simulink model "REL"  (R2022a)
settings: Solver=FixedStepDiscrete  StartTime=0.0  StopTime=10.0  FixedStep=0.01  RelTol=1e-3
libraries: simulink x4, DoorRatSts x4, DoorRlsDriver x2, DoorRlsReq x2
settings Model: Creator=DELL  LastModifiedBy=DELL
settings DataIOCC: SaveFormat=StructureWithTime
settings OptimizationCC: DefaultParameterBehavior=Inlined  EnhancedBackFolding=on  PassReuseOutputArgsAs=Individual arguments  ZeroExternalMemoryAtStartup=off  ZeroInternalMemoryAtStartup=off  OptimizeBlockOrder=speed  DifferentSizesBufferReuse=on  OptimizationCustomize=off  EfficientTunableParamExpr=on
settings DebuggingCC: ParameterTunabilityLossMsg=error
settings ModelReferenceCC: ModelReferenceNumInstancesAllowed=Single
settings SFSimCC: MATLABDynamicMemAlloc=off
settings RTWCC: Description=AUTOSAR  SystemTargetFile=autosar.tlc  GenCodeOnly=on  TemplateMakefile=ert_default_tmf
settings CodeAppCC: ForceParamTrailComments=on  IgnoreCustomStorageClasses=off  OperatorAnnotations=on  SimulinkDataObjDesc=on  SFDataObjDesc=on  InsertBlockDesc=on
settings STFCustomTargetCC: TargetLangStandard=C99 (ISO)  MultiwordLength=256  ParMdlRefBuildCompliant=on  CompOptLevelCompliant=on  IncludeMdlTerminateFcn=off  CombineOutputUpdateFcns=on  SuppressErrorStatus=on  ERTCustomFileBanners=on  SupportNonFinite=off  SupportComplex=off  SupportContinuousTime=off  SupportNonInlinedSFcns=off  RemoveResetFunc=on  MATLABClassNameForMDSCustomization=Simulink.SoftwareTarget.ERTCustomization  AutosarCompliant=on  GRTInterface=off  UseToolchainInfoCompliant=on  LookupTableObjectStructAxisOrder=2,1,3,4,...  LUTObjectStructOrderEvenSpacing=Size,Table,Breakpoints  SystemTargetFile=autosar.tlc
settings ERTTargetCC: TargetLangStandard=C99 (ISO)  ConcurrentExecutionCompliant=off  IncludeMdlTerminateFcn=off  SuppressErrorStatus=on  SupportNonFinite=off  SupportComplex=off  ModelStepFunctionPrototypeControlCompliant=off  CPPClassGenCompliant=off  AutosarCompliant=on  LookupTableObjectStructAxisOrder=2,1,3,4,...  LUTObjectStructOrderEvenSpacing=Size,Table,Breakpoints  InlinedParameterPlacement=NonHierarchical  ERTCustomFileTemplate=example_file_process.tlc

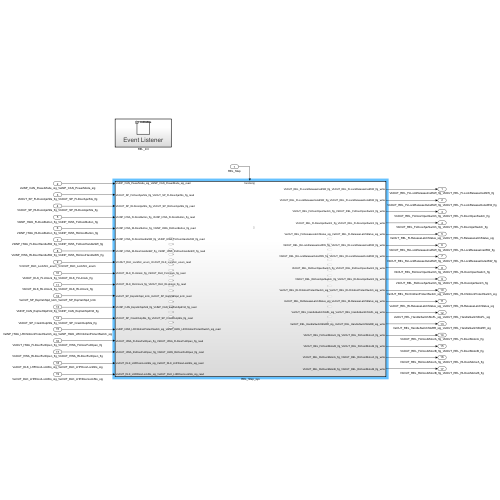
[thumbnail: Simulink's stored preview of the top-level diagram]
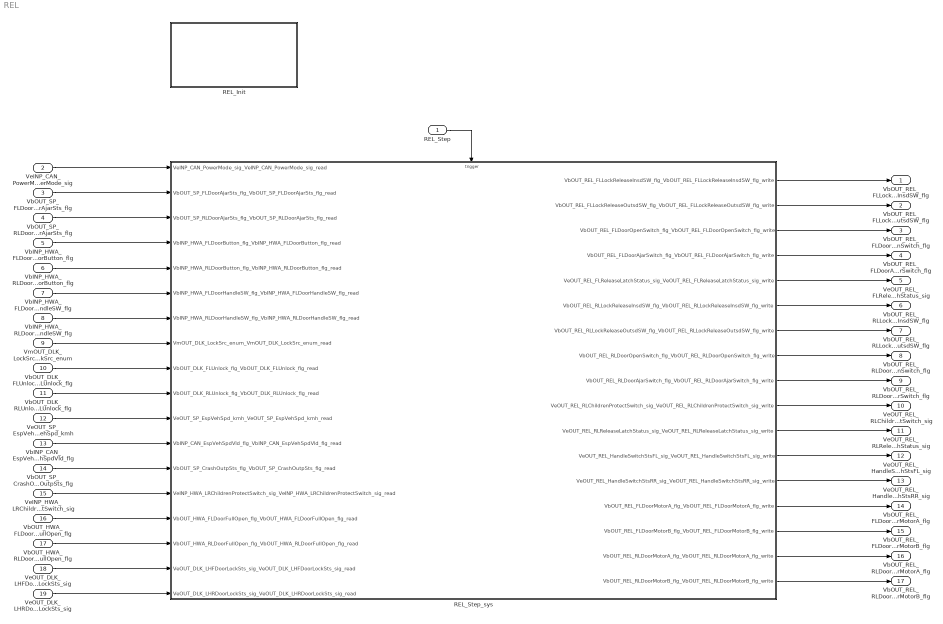
== system REL ==
  REL_Step : Inport  SampleTime=0.01  OutputFunctionCall=on
  VeINP_CAN_PowerMode_sig_VeINP_CAN_PowerMode_sig : Inport  Port=2  OutDataTypeStr=UInt8  PortDimensions=1
  VbOUT_SP_FLDoorAjarSts_flg_VbOUT_SP_FLDoorAjarSts_flg : Inport  Port=3  OutDataTypeStr=Boolean  PortDimensions=1
  VbOUT_SP_RLDoorAjarSts_flg_VbOUT_SP_RLDoorAjarSts_flg : Inport  Port=4  OutDataTypeStr=Boolean  PortDimensions=1
  VbINP_HWA_FLDoorButton_flg_VbINP_HWA_FLDoorButton_flg : Inport  Port=5  OutDataTypeStr=Boolean  PortDimensions=1
  VbINP_HWA_RLDoorButton_flg_VbINP_HWA_RLDoorButton_flg : Inport  Port=6  OutDataTypeStr=Boolean  PortDimensions=1
  VbINP_HWA_FLDoorHandleSW_flg_VbINP_HWA_FLDoorHandleSW_flg : Inport  Port=7  OutDataTypeStr=Boolean  PortDimensions=1
  VbINP_HWA_RLDoorHandleSW_flg_VbINP_HWA_RLDoorHandleSW_flg : Inport  Port=8  OutDataTypeStr=Boolean  PortDimensions=1
  VmOUT_DLK_LockSrc_enum_VmOUT_DLK_LockSrc_enum : Inport  Port=9  OutDataTypeStr=UInt8  PortDimensions=1
  VbOUT_DLK_FLUnlock_flg_VbOUT_DLK_FLUnlock_flg : Inport  Port=10  OutDataTypeStr=Boolean  PortDimensions=1
  VbOUT_DLK_RLUnlock_flg_VbOUT_DLK_RLUnlock_flg : Inport  Port=11  OutDataTypeStr=Boolean  PortDimensions=1
  VeOUT_SP_EspVehSpd_kmh_VeOUT_SP_EspVehSpd_kmh : Inport  Port=12  OutDataTypeStr=UInt8  PortDimensions=1
  VbINP_CAN_EspVehSpdVld_flg_VbINP_CAN_EspVehSpdVld_flg : Inport  Port=13  OutDataTypeStr=Boolean  PortDimensions=1
  VbOUT_SP_CrashOutpSts_flg_VbOUT_SP_CrashOutpSts_flg : Inport  Port=14  OutDataTypeStr=Boolean  PortDimensions=1
  VeINP_HWA_LRChildrenProtectSwitch_sig_VeINP_HWA_LRChildrenProtectSwitch_sig : Inport  Port=15  OutDataTypeStr=UInt8  PortDimensions=1
  VbOUT_HWA_FLDoorFullOpen_flg_VbOUT_HWA_FLDoorFullOpen_flg : Inport  Port=16  OutDataTypeStr=Boolean  PortDimensions=1
  VbOUT_HWA_RLDoorFullOpen_flg_VbOUT_HWA_RLDoorFullOpen_flg : Inport  Port=17  OutDataTypeStr=Boolean  PortDimensions=1
  VeOUT_DLK_LHFDoorLockSts_sig_VeOUT_DLK_LHFDoorLockSts_sig : Inport  Port=18  OutDataTypeStr=UInt8  PortDimensions=1
  VeOUT_DLK_LHRDoorLockSts_sig_VeOUT_DLK_LHRDoorLockSts_sig : Inport  Port=19  OutDataTypeStr=UInt8  PortDimensions=1
  REL_Init : Subsystem
  REL_Step_sys : Subsystem
  VbOUT_REL_FLLockReleaseInsdSW_flg_VbOUT_REL_FLLockReleaseInsdSW_flg : Outport  OutDataTypeStr=Boolean  PortDimensions=1
  VbOUT_REL_FLLockReleaseOutsdSW_flg_VbOUT_REL_FLLockReleaseOutsdSW_flg : Outport  Port=2  OutDataTypeStr=Boolean  PortDimensions=1
  VbOUT_REL_FLDoorOpenSwitch_flg_VbOUT_REL_FLDoorOpenSwitch_flg : Outport  Port=3  OutDataTypeStr=Boolean  PortDimensions=1
  VbOUT_REL_FLDoorAjarSwitch_flg_VbOUT_REL_FLDoorAjarSwitch_flg : Outport  Port=4  OutDataTypeStr=Boolean  PortDimensions=1
  VeOUT_REL_FLReleaseLatchStatus_sig_VeOUT_REL_FLReleaseLatchStatus_sig : Outport  Port=5  OutDataTypeStr=UInt8  PortDimensions=1
  VbOUT_REL_RLLockReleaseInsdSW_flg_VbOUT_REL_RLLockReleaseInsdSW_flg : Outport  Port=6  OutDataTypeStr=Boolean  PortDimensions=1
  VbOUT_REL_RLLockReleaseOutsdSW_flg_VbOUT_REL_RLLockReleaseOutsdSW_flg : Outport  Port=7  OutDataTypeStr=Boolean  PortDimensions=1
  VbOUT_REL_RLDoorOpenSwitch_flg_VbOUT_REL_RLDoorOpenSwitch_flg : Outport  Port=8  OutDataTypeStr=Boolean  PortDimensions=1
  VbOUT_REL_RLDoorAjarSwitch_flg_VbOUT_REL_RLDoorAjarSwitch_flg : Outport  Port=9  OutDataTypeStr=Boolean  PortDimensions=1
  VeOUT_REL_RLChildrenProtectSwitch_sig_VeOUT_REL_RLChildrenProtectSwitch_sig : Outport  Port=10  OutDataTypeStr=UInt8  PortDimensions=1
  VeOUT_REL_RLReleaseLatchStatus_sig_VeOUT_REL_RLReleaseLatchStatus_sig : Outport  Port=11  OutDataTypeStr=UInt8  PortDimensions=1
  VeOUT_REL_HandleSwitchStsFL_sig_VeOUT_REL_HandleSwitchStsFL_sig : Outport  Port=12  OutDataTypeStr=UInt8  PortDimensions=1
  VeOUT_REL_HandleSwitchStsRR_sig_VeOUT_REL_HandleSwitchStsRR_sig : Outport  Port=13  OutDataTypeStr=UInt8  PortDimensions=1
  VbOUT_REL_FLDoorMotorA_flg_VbOUT_REL_FLDoorMotorA_flg : Outport  Port=14  OutDataTypeStr=Boolean  PortDimensions=1
  VbOUT_REL_FLDoorMotorB_flg_VbOUT_REL_FLDoorMotorB_flg : Outport  Port=15  OutDataTypeStr=Boolean  PortDimensions=1
  VbOUT_REL_RLDoorMotorA_flg_VbOUT_REL_RLDoorMotorA_flg : Outport  Port=16  OutDataTypeStr=Boolean  PortDimensions=1
  VbOUT_REL_RLDoorMotorB_flg_VbOUT_REL_RLDoorMotorB_flg : Outport  Port=17  OutDataTypeStr=Boolean  PortDimensions=1
  wires:
  VeINP_CAN_PowerMode_sig_VeINP_CAN_PowerMode_sig/1 -> REL_Step_sys/1(VeINP_CAN_PowerMode_sig_VeINP_CAN_PowerMode_sig_read)
  VbOUT_SP_FLDoorAjarSts_flg_VbOUT_SP_FLDoorAjarSts_flg/1 -> REL_Step_sys/2(VbOUT_SP_FLDoorAjarSts_flg_VbOUT_SP_FLDoorAjarSts_flg_read)
  VbOUT_SP_RLDoorAjarSts_flg_VbOUT_SP_RLDoorAjarSts_flg/1 -> REL_Step_sys/3(VbOUT_SP_RLDoorAjarSts_flg_VbOUT_SP_RLDoorAjarSts_flg_read)
  VbINP_HWA_FLDoorButton_flg_VbINP_HWA_FLDoorButton_flg/1 -> REL_Step_sys/4(VbINP_HWA_FLDoorButton_flg_VbINP_HWA_FLDoorButton_flg_read)
  VbINP_HWA_RLDoorButton_flg_VbINP_HWA_RLDoorButton_flg/1 -> REL_Step_sys/5(VbINP_HWA_RLDoorButton_flg_VbINP_HWA_RLDoorButton_flg_read)
  VbINP_HWA_FLDoorHandleSW_flg_VbINP_HWA_FLDoorHandleSW_flg/1 -> REL_Step_sys/6(VbINP_HWA_FLDoorHandleSW_flg_VbINP_HWA_FLDoorHandleSW_flg_read)
  VbINP_HWA_RLDoorHandleSW_flg_VbINP_HWA_RLDoorHandleSW_flg/1 -> REL_Step_sys/7(VbINP_HWA_RLDoorHandleSW_flg_VbINP_HWA_RLDoorHandleSW_flg_read)
  VmOUT_DLK_LockSrc_enum_VmOUT_DLK_LockSrc_enum/1 -> REL_Step_sys/8(VmOUT_DLK_LockSrc_enum_VmOUT_DLK_LockSrc_enum_read)
  VbOUT_DLK_FLUnlock_flg_VbOUT_DLK_FLUnlock_flg/1 -> REL_Step_sys/9(VbOUT_DLK_FLUnlock_flg_VbOUT_DLK_FLUnlock_flg_read)
  VbOUT_DLK_RLUnlock_flg_VbOUT_DLK_RLUnlock_flg/1 -> REL_Step_sys/10(VbOUT_DLK_RLUnlock_flg_VbOUT_DLK_RLUnlock_flg_read)
  VeOUT_SP_EspVehSpd_kmh_VeOUT_SP_EspVehSpd_kmh/1 -> REL_Step_sys/11(VeOUT_SP_EspVehSpd_kmh_VeOUT_SP_EspVehSpd_kmh_read)
  VbINP_CAN_EspVehSpdVld_flg_VbINP_CAN_EspVehSpdVld_flg/1 -> REL_Step_sys/12(VbINP_CAN_EspVehSpdVld_flg_VbINP_CAN_EspVehSpdVld_flg_read)
  VbOUT_SP_CrashOutpSts_flg_VbOUT_SP_CrashOutpSts_flg/1 -> REL_Step_sys/13(VbOUT_SP_CrashOutpSts_flg_VbOUT_SP_CrashOutpSts_flg_read)
  VeINP_HWA_LRChildrenProtectSwitch_sig_VeINP_HWA_LRChildrenProtectSwitch_sig/1 -> REL_Step_sys/14(VeINP_HWA_LRChildrenProtectSwitch_sig_VeINP_HWA_LRChildrenProtectSwitch_sig_read)
  VbOUT_HWA_FLDoorFullOpen_flg_VbOUT_HWA_FLDoorFullOpen_flg/1 -> REL_Step_sys/15(VbOUT_HWA_FLDoorFullOpen_flg_VbOUT_HWA_FLDoorFullOpen_flg_read)
  VbOUT_HWA_RLDoorFullOpen_flg_VbOUT_HWA_RLDoorFullOpen_flg/1 -> REL_Step_sys/16(VbOUT_HWA_RLDoorFullOpen_flg_VbOUT_HWA_RLDoorFullOpen_flg_read)
  VeOUT_DLK_LHFDoorLockSts_sig_VeOUT_DLK_LHFDoorLockSts_sig/1 -> REL_Step_sys/17(VeOUT_DLK_LHFDoorLockSts_sig_VeOUT_DLK_LHFDoorLockSts_sig_read)
  VeOUT_DLK_LHRDoorLockSts_sig_VeOUT_DLK_LHRDoorLockSts_sig/1 -> REL_Step_sys/18(VeOUT_DLK_LHRDoorLockSts_sig_VeOUT_DLK_LHRDoorLockSts_sig_read)
  REL_Step_sys/1(VbOUT_REL_FLLockReleaseInsdSW_flg_VbOUT_REL_FLLockReleaseInsdSW_flg_write) -> VbOUT_REL_FLLockReleaseInsdSW_flg_VbOUT_REL_FLLockReleaseInsdSW_flg/1
  REL_Step_sys/2(VbOUT_REL_FLLockReleaseOutsdSW_flg_VbOUT_REL_FLLockReleaseOutsdSW_flg_write) -> VbOUT_REL_FLLockReleaseOutsdSW_flg_VbOUT_REL_FLLockReleaseOutsdSW_flg/1
  REL_Step_sys/3(VbOUT_REL_FLDoorOpenSwitch_flg_VbOUT_REL_FLDoorOpenSwitch_flg_write) -> VbOUT_REL_FLDoorOpenSwitch_flg_VbOUT_REL_FLDoorOpenSwitch_flg/1
  REL_Step_sys/4(VbOUT_REL_FLDoorAjarSwitch_flg_VbOUT_REL_FLDoorAjarSwitch_flg_write) -> VbOUT_REL_FLDoorAjarSwitch_flg_VbOUT_REL_FLDoorAjarSwitch_flg/1
  REL_Step_sys/5(VeOUT_REL_FLReleaseLatchStatus_sig_VeOUT_REL_FLReleaseLatchStatus_sig_write) -> VeOUT_REL_FLReleaseLatchStatus_sig_VeOUT_REL_FLReleaseLatchStatus_sig/1
  REL_Step_sys/6(VbOUT_REL_RLLockReleaseInsdSW_flg_VbOUT_REL_RLLockReleaseInsdSW_flg_write) -> VbOUT_REL_RLLockReleaseInsdSW_flg_VbOUT_REL_RLLockReleaseInsdSW_flg/1
  REL_Step_sys/7(VbOUT_REL_RLLockReleaseOutsdSW_flg_VbOUT_REL_RLLockReleaseOutsdSW_flg_write) -> VbOUT_REL_RLLockReleaseOutsdSW_flg_VbOUT_REL_RLLockReleaseOutsdSW_flg/1
  REL_Step_sys/8(VbOUT_REL_RLDoorOpenSwitch_flg_VbOUT_REL_RLDoorOpenSwitch_flg_write) -> VbOUT_REL_RLDoorOpenSwitch_flg_VbOUT_REL_RLDoorOpenSwitch_flg/1
  REL_Step_sys/9(VbOUT_REL_RLDoorAjarSwitch_flg_VbOUT_REL_RLDoorAjarSwitch_flg_write) -> VbOUT_REL_RLDoorAjarSwitch_flg_VbOUT_REL_RLDoorAjarSwitch_flg/1
  REL_Step_sys/10(VeOUT_REL_RLChildrenProtectSwitch_sig_VeOUT_REL_RLChildrenProtectSwitch_sig_write) -> VeOUT_REL_RLChildrenProtectSwitch_sig_VeOUT_REL_RLChildrenProtectSwitch_sig/1
  REL_Step_sys/11(VeOUT_REL_RLReleaseLatchStatus_sig_VeOUT_REL_RLReleaseLatchStatus_sig_write) -> VeOUT_REL_RLReleaseLatchStatus_sig_VeOUT_REL_RLReleaseLatchStatus_sig/1
  REL_Step_sys/12(VeOUT_REL_HandleSwitchStsFL_sig_VeOUT_REL_HandleSwitchStsFL_sig_write) -> VeOUT_REL_HandleSwitchStsFL_sig_VeOUT_REL_HandleSwitchStsFL_sig/1
  REL_Step_sys/13(VeOUT_REL_HandleSwitchStsRR_sig_VeOUT_REL_HandleSwitchStsRR_sig_write) -> VeOUT_REL_HandleSwitchStsRR_sig_VeOUT_REL_HandleSwitchStsRR_sig/1
  REL_Step_sys/14(VbOUT_REL_FLDoorMotorA_flg_VbOUT_REL_FLDoorMotorA_flg_write) -> VbOUT_REL_FLDoorMotorA_flg_VbOUT_REL_FLDoorMotorA_flg/1
  REL_Step_sys/15(VbOUT_REL_FLDoorMotorB_flg_VbOUT_REL_FLDoorMotorB_flg_write) -> VbOUT_REL_FLDoorMotorB_flg_VbOUT_REL_FLDoorMotorB_flg/1
  REL_Step_sys/16(VbOUT_REL_RLDoorMotorA_flg_VbOUT_REL_RLDoorMotorA_flg_write) -> VbOUT_REL_RLDoorMotorA_flg_VbOUT_REL_RLDoorMotorA_flg/1
  REL_Step_sys/17(VbOUT_REL_RLDoorMotorB_flg_VbOUT_REL_RLDoorMotorB_flg_write) -> VbOUT_REL_RLDoorMotorB_flg_VbOUT_REL_RLDoorMotorB_flg/1
  REL_Step/1 -> REL_Step_sys/Trigger

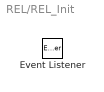
== system REL/REL_Init ==
  Event Listener : EventListener  EventName=reset

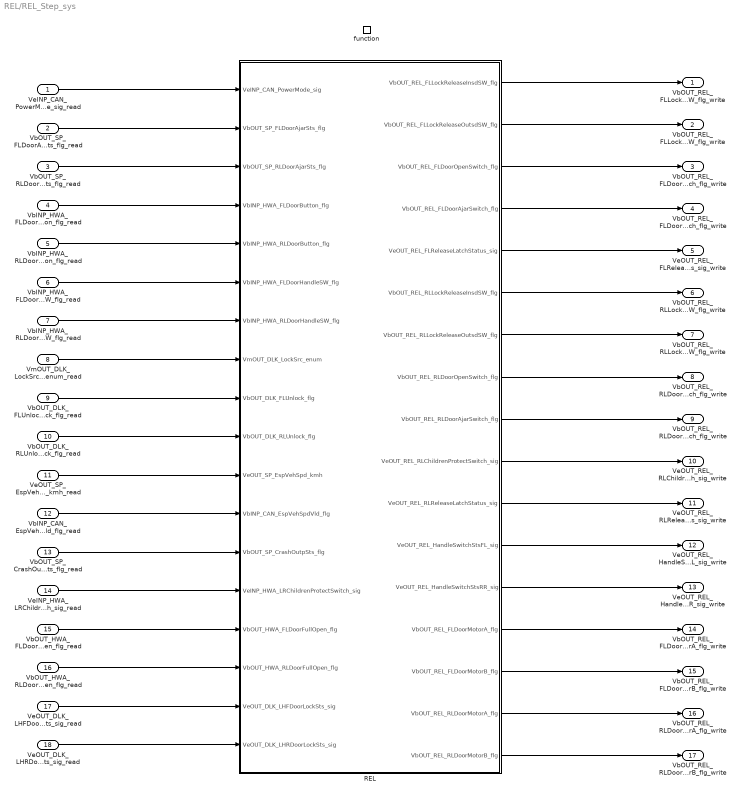
== system REL/REL_Step_sys ==
  VeINP_CAN_PowerMode_sig_VeINP_CAN_PowerMode_sig_read : Inport
  VbOUT_SP_FLDoorAjarSts_flg_VbOUT_SP_FLDoorAjarSts_flg_read : Inport  Port=2
  VbOUT_SP_RLDoorAjarSts_flg_VbOUT_SP_RLDoorAjarSts_flg_read : Inport  Port=3
  VbINP_HWA_FLDoorButton_flg_VbINP_HWA_FLDoorButton_flg_read : Inport  Port=4
  VbINP_HWA_RLDoorButton_flg_VbINP_HWA_RLDoorButton_flg_read : Inport  Port=5
  VbINP_HWA_FLDoorHandleSW_flg_VbINP_HWA_FLDoorHandleSW_flg_read : Inport  Port=6
  VbINP_HWA_RLDoorHandleSW_flg_VbINP_HWA_RLDoorHandleSW_flg_read : Inport  Port=7
  VmOUT_DLK_LockSrc_enum_VmOUT_DLK_LockSrc_enum_read : Inport  Port=8
  VbOUT_DLK_FLUnlock_flg_VbOUT_DLK_FLUnlock_flg_read : Inport  Port=9
  VbOUT_DLK_RLUnlock_flg_VbOUT_DLK_RLUnlock_flg_read : Inport  Port=10
  VeOUT_SP_EspVehSpd_kmh_VeOUT_SP_EspVehSpd_kmh_read : Inport  Port=11
  VbINP_CAN_EspVehSpdVld_flg_VbINP_CAN_EspVehSpdVld_flg_read : Inport  Port=12
  VbOUT_SP_CrashOutpSts_flg_VbOUT_SP_CrashOutpSts_flg_read : Inport  Port=13
  VeINP_HWA_LRChildrenProtectSwitch_sig_VeINP_HWA_LRChildrenProtectSwitch_sig_read : Inport  Port=14
  VbOUT_HWA_FLDoorFullOpen_flg_VbOUT_HWA_FLDoorFullOpen_flg_read : Inport  Port=15
  VbOUT_HWA_RLDoorFullOpen_flg_VbOUT_HWA_RLDoorFullOpen_flg_read : Inport  Port=16
  VeOUT_DLK_LHFDoorLockSts_sig_VeOUT_DLK_LHFDoorLockSts_sig_read : Inport  Port=17
  VeOUT_DLK_LHRDoorLockSts_sig_VeOUT_DLK_LHRDoorLockSts_sig_read : Inport  Port=18
  function : TriggerPort  TriggerType=function-call  VariantControl=(inherit)  SampleTimeType=periodic  SampleTime=-1
  REL : Subsystem
  VbOUT_REL_FLLockReleaseInsdSW_flg_VbOUT_REL_FLLockReleaseInsdSW_flg_write : Outport
      settings: EnsureOutportIsVirtual=on
  VbOUT_REL_FLLockReleaseOutsdSW_flg_VbOUT_REL_FLLockReleaseOutsdSW_flg_write : Outport  Port=2
      settings: EnsureOutportIsVirtual=on
  VbOUT_REL_FLDoorOpenSwitch_flg_VbOUT_REL_FLDoorOpenSwitch_flg_write : Outport  Port=3
      settings: EnsureOutportIsVirtual=on
  VbOUT_REL_FLDoorAjarSwitch_flg_VbOUT_REL_FLDoorAjarSwitch_flg_write : Outport  Port=4
      settings: EnsureOutportIsVirtual=on
  VeOUT_REL_FLReleaseLatchStatus_sig_VeOUT_REL_FLReleaseLatchStatus_sig_write : Outport  Port=5
      settings: EnsureOutportIsVirtual=on
  VbOUT_REL_RLLockReleaseInsdSW_flg_VbOUT_REL_RLLockReleaseInsdSW_flg_write : Outport  Port=6
      settings: EnsureOutportIsVirtual=on
  VbOUT_REL_RLLockReleaseOutsdSW_flg_VbOUT_REL_RLLockReleaseOutsdSW_flg_write : Outport  Port=7
      settings: EnsureOutportIsVirtual=on
  VbOUT_REL_RLDoorOpenSwitch_flg_VbOUT_REL_RLDoorOpenSwitch_flg_write : Outport  Port=8
      settings: EnsureOutportIsVirtual=on
  VbOUT_REL_RLDoorAjarSwitch_flg_VbOUT_REL_RLDoorAjarSwitch_flg_write : Outport  Port=9
      settings: EnsureOutportIsVirtual=on
  VeOUT_REL_RLChildrenProtectSwitch_sig_VeOUT_REL_RLChildrenProtectSwitch_sig_write : Outport  Port=10
      settings: EnsureOutportIsVirtual=on
  VeOUT_REL_RLReleaseLatchStatus_sig_VeOUT_REL_RLReleaseLatchStatus_sig_write : Outport  Port=11
      settings: EnsureOutportIsVirtual=on
  VeOUT_REL_HandleSwitchStsFL_sig_VeOUT_REL_HandleSwitchStsFL_sig_write : Outport  Port=12
      settings: EnsureOutportIsVirtual=on
  VeOUT_REL_HandleSwitchStsRR_sig_VeOUT_REL_HandleSwitchStsRR_sig_write : Outport  Port=13
      settings: EnsureOutportIsVirtual=on
  VbOUT_REL_FLDoorMotorA_flg_VbOUT_REL_FLDoorMotorA_flg_write : Outport  Port=14
      settings: EnsureOutportIsVirtual=on
  VbOUT_REL_FLDoorMotorB_flg_VbOUT_REL_FLDoorMotorB_flg_write : Outport  Port=15
      settings: EnsureOutportIsVirtual=on
  VbOUT_REL_RLDoorMotorA_flg_VbOUT_REL_RLDoorMotorA_flg_write : Outport  Port=16
      settings: EnsureOutportIsVirtual=on
  VbOUT_REL_RLDoorMotorB_flg_VbOUT_REL_RLDoorMotorB_flg_write : Outport  Port=17
      settings: EnsureOutportIsVirtual=on
  wires:
  REL/1(VbOUT_REL_FLLockReleaseInsdSW_flg) -> VbOUT_REL_FLLockReleaseInsdSW_flg_VbOUT_REL_FLLockReleaseInsdSW_flg_write/1
  REL/2(VbOUT_REL_FLLockReleaseOutsdSW_flg) -> VbOUT_REL_FLLockReleaseOutsdSW_flg_VbOUT_REL_FLLockReleaseOutsdSW_flg_write/1
  REL/3(VbOUT_REL_FLDoorOpenSwitch_flg) -> VbOUT_REL_FLDoorOpenSwitch_flg_VbOUT_REL_FLDoorOpenSwitch_flg_write/1
  REL/4(VbOUT_REL_FLDoorAjarSwitch_flg) -> VbOUT_REL_FLDoorAjarSwitch_flg_VbOUT_REL_FLDoorAjarSwitch_flg_write/1
  REL/5(VeOUT_REL_FLReleaseLatchStatus_sig) -> VeOUT_REL_FLReleaseLatchStatus_sig_VeOUT_REL_FLReleaseLatchStatus_sig_write/1
  REL/6(VbOUT_REL_RLLockReleaseInsdSW_flg) -> VbOUT_REL_RLLockReleaseInsdSW_flg_VbOUT_REL_RLLockReleaseInsdSW_flg_write/1
  REL/7(VbOUT_REL_RLLockReleaseOutsdSW_flg) -> VbOUT_REL_RLLockReleaseOutsdSW_flg_VbOUT_REL_RLLockReleaseOutsdSW_flg_write/1
  REL/8(VbOUT_REL_RLDoorOpenSwitch_flg) -> VbOUT_REL_RLDoorOpenSwitch_flg_VbOUT_REL_RLDoorOpenSwitch_flg_write/1
  REL/9(VbOUT_REL_RLDoorAjarSwitch_flg) -> VbOUT_REL_RLDoorAjarSwitch_flg_VbOUT_REL_RLDoorAjarSwitch_flg_write/1
  REL/10(VeOUT_REL_RLChildrenProtectSwitch_sig) -> VeOUT_REL_RLChildrenProtectSwitch_sig_VeOUT_REL_RLChildrenProtectSwitch_sig_write/1
  REL/11(VeOUT_REL_RLReleaseLatchStatus_sig) -> VeOUT_REL_RLReleaseLatchStatus_sig_VeOUT_REL_RLReleaseLatchStatus_sig_write/1
  REL/12(VeOUT_REL_HandleSwitchStsFL_sig) -> VeOUT_REL_HandleSwitchStsFL_sig_VeOUT_REL_HandleSwitchStsFL_sig_write/1
  REL/13(VeOUT_REL_HandleSwitchStsRR_sig) -> VeOUT_REL_HandleSwitchStsRR_sig_VeOUT_REL_HandleSwitchStsRR_sig_write/1
  REL/14(VbOUT_REL_FLDoorMotorA_flg) -> VbOUT_REL_FLDoorMotorA_flg_VbOUT_REL_FLDoorMotorA_flg_write/1
  REL/15(VbOUT_REL_FLDoorMotorB_flg) -> VbOUT_REL_FLDoorMotorB_flg_VbOUT_REL_FLDoorMotorB_flg_write/1
  REL/16(VbOUT_REL_RLDoorMotorA_flg) -> VbOUT_REL_RLDoorMotorA_flg_VbOUT_REL_RLDoorMotorA_flg_write/1
  REL/17(VbOUT_REL_RLDoorMotorB_flg) -> VbOUT_REL_RLDoorMotorB_flg_VbOUT_REL_RLDoorMotorB_flg_write/1
  VeINP_CAN_PowerMode_sig_VeINP_CAN_PowerMode_sig_read/1 -> REL/1(VeINP_CAN_PowerMode_sig)
  VbOUT_SP_FLDoorAjarSts_flg_VbOUT_SP_FLDoorAjarSts_flg_read/1 -> REL/2(VbOUT_SP_FLDoorAjarSts_flg)
  VbOUT_SP_RLDoorAjarSts_flg_VbOUT_SP_RLDoorAjarSts_flg_read/1 -> REL/3(VbOUT_SP_RLDoorAjarSts_flg)
  VbINP_HWA_FLDoorButton_flg_VbINP_HWA_FLDoorButton_flg_read/1 -> REL/4(VbINP_HWA_FLDoorButton_flg)
  VbINP_HWA_RLDoorButton_flg_VbINP_HWA_RLDoorButton_flg_read/1 -> REL/5(VbINP_HWA_RLDoorButton_flg)
  VbINP_HWA_FLDoorHandleSW_flg_VbINP_HWA_FLDoorHandleSW_flg_read/1 -> REL/6(VbINP_HWA_FLDoorHandleSW_flg)
  VbINP_HWA_RLDoorHandleSW_flg_VbINP_HWA_RLDoorHandleSW_flg_read/1 -> REL/7(VbINP_HWA_RLDoorHandleSW_flg)
  VmOUT_DLK_LockSrc_enum_VmOUT_DLK_LockSrc_enum_read/1 -> REL/8(VmOUT_DLK_LockSrc_enum)
  VbOUT_DLK_FLUnlock_flg_VbOUT_DLK_FLUnlock_flg_read/1 -> REL/9(VbOUT_DLK_FLUnlock_flg)
  VbOUT_DLK_RLUnlock_flg_VbOUT_DLK_RLUnlock_flg_read/1 -> REL/10(VbOUT_DLK_RLUnlock_flg)
  VeOUT_SP_EspVehSpd_kmh_VeOUT_SP_EspVehSpd_kmh_read/1 -> REL/11(VeOUT_SP_EspVehSpd_kmh)
  VbINP_CAN_EspVehSpdVld_flg_VbINP_CAN_EspVehSpdVld_flg_read/1 -> REL/12(VbINP_CAN_EspVehSpdVld_flg)
  VbOUT_SP_CrashOutpSts_flg_VbOUT_SP_CrashOutpSts_flg_read/1 -> REL/13(VbOUT_SP_CrashOutpSts_flg)
  VeINP_HWA_LRChildrenProtectSwitch_sig_VeINP_HWA_LRChildrenProtectSwitch_sig_read/1 -> REL/14(VeINP_HWA_LRChildrenProtectSwitch_sig)
  VbOUT_HWA_FLDoorFullOpen_flg_VbOUT_HWA_FLDoorFullOpen_flg_read/1 -> REL/15(VbOUT_HWA_FLDoorFullOpen_flg)
  VbOUT_HWA_RLDoorFullOpen_flg_VbOUT_HWA_RLDoorFullOpen_flg_read/1 -> REL/16(VbOUT_HWA_RLDoorFullOpen_flg)
  VeOUT_DLK_LHFDoorLockSts_sig_VeOUT_DLK_LHFDoorLockSts_sig_read/1 -> REL/17(VeOUT_DLK_LHFDoorLockSts_sig)
  VeOUT_DLK_LHRDoorLockSts_sig_VeOUT_DLK_LHRDoorLockSts_sig_read/1 -> REL/18(VeOUT_DLK_LHRDoorLockSts_sig)

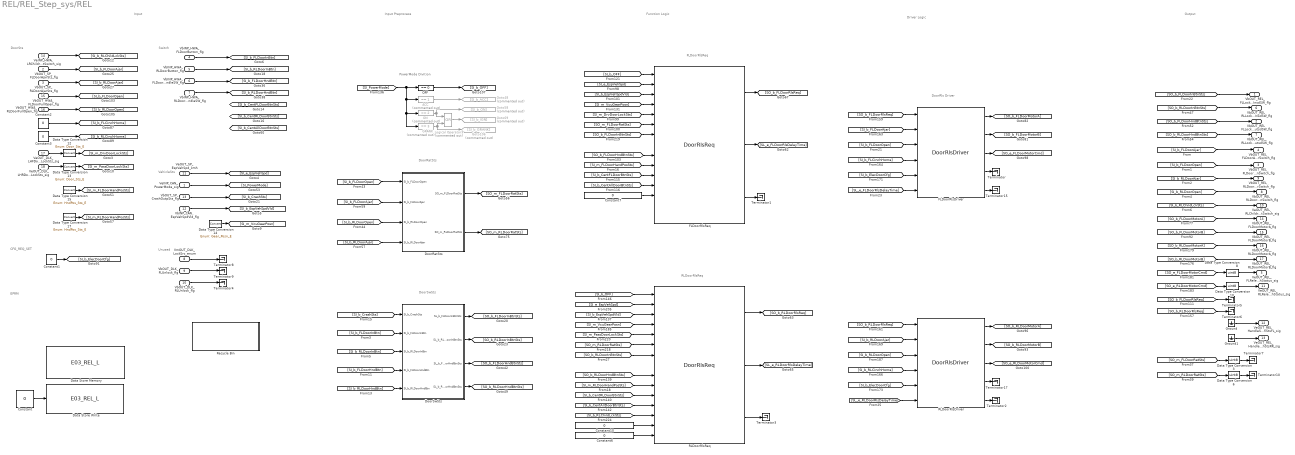
== system REL/REL_Step_sys/REL ==
  note: VehicleSts
  note: Function Logic
  note: Input
  note: Output
  note: Input Preprocess
  note: EPRM
  note: PowerMode Divition
  note: DoorRatSts
  note: Driver Logic
  note: DoorRls Driver
  note: FLDoorRlsReq
  note: RLDoorRlsReq
  note: DoorSwSts
  note: Switch
  note: DoorSts
  note: CFG_REQ_SET
  note: Unused
  VeINP_CAN_PowerMode_sig : Inport
  VbOUT_SP_FLDoorAjarSts_flg : Inport  Port=2
  VbOUT_SP_RLDoorAjarSts_flg : Inport  Port=3
  VbINP_HWA_FLDoorButton_flg : Inport  Port=4
  VbINP_HWA_RLDoorButton_flg : Inport  Port=5
  VbINP_HWA_FLDoorHandleSW_flg : Inport  Port=6
  VbINP_HWA_RLDoorHandleSW_flg : Inport  Port=7
  VmOUT_DLK_LockSrc_enum : Inport  Port=8
  VbOUT_DLK_FLUnlock_flg : Inport  Port=9
  VbOUT_DLK_RLUnlock_flg : Inport  Port=10
  VeOUT_SP_EspVehSpd_kmh : Inport  Port=11
  VbINP_CAN_EspVehSpdVld_flg : Inport  Port=12
  VbOUT_SP_CrashOutpSts_flg : Inport  Port=13
  VeINP_HWA_LRChildrenProtectSwitch_sig : Inport  Port=14
  VbOUT_HWA_FLDoorFullOpen_flg : Inport  Port=15
  VbOUT_HWA_RLDoorFullOpen_flg : Inport  Port=16
  VeOUT_DLK_LHFDoorLockSts_sig : Inport  Port=17
  VeOUT_DLK_LHRDoorLockSts_sig : Inport  Port=18
  ACC : simulink/Logic and Bit Operations/Compare To Constant  Commented=on  relop===  const=1  OutDataTypeStr=boolean
  Constant : Constant  Value=0  OutDataTypeStr=uint8
  Constant{1..3,6..7,10} (6 alike) : Constant  Value=0  OutDataTypeStr=boolean
  Data Store Memory : DataStoreMemory  DataStoreName=E03_REL_L  WriteAfterWriteMsg=warning  ShowAdditionalParam=off  OutDataTypeStr=uint8
  Data Store Write : DataStoreWrite  DataStoreName=E03_REL_L  IndexOptions=Index vector (dialog)  Indices=1  OutputSizes=1
  Data Type Conversion{3,6,8,10} (4 alike) : DataTypeConversion  OutDataTypeStr=uint8  SaturateOnIntegerOverflow=off  RndMeth=Floor
  Data Type Conversion12 : DataTypeConversion  OutDataTypeStr=Enum: Door_Sts_E  SaturateOnIntegerOverflow=off  RndMeth=Floor
  Data Type Conversion13 : DataTypeConversion  OutDataTypeStr=Enum: Door_Sts_E  SaturateOnIntegerOverflow=off  RndMeth=Floor
  Data Type Conversion14 : DataTypeConversion  OutDataTypeStr=Enum: Gear_Posn_E  SaturateOnIntegerOverflow=off  RndMeth=Floor
  Data Type Conversion15 : DataTypeConversion  OutDataTypeStr=Enum: HndPos_Sts_E  SaturateOnIntegerOverflow=off  RndMeth=Floor
  Data Type Conversion17 : DataTypeConversion  OutDataTypeStr=Enum: HndPos_Sts_E  SaturateOnIntegerOverflow=off  RndMeth=Floor
  DoorRatSts : Stateflow chart  TreatAsAtomicUnit=on
  DoorSwSts : Stateflow chart  TreatAsAtomicUnit=on
  FLDoorRlsDriver : DoorRlsDriver/DoorRlsDriver  SystemSampleTime=-1  VariantActivationTime=update diagram  Latency=0  AutoFrameSizeCalculation=off
  FLDoorRlsReq : DoorRlsReq/DoorRlsReq  SystemSampleTime=-1  VariantActivationTime=update diagram  Latency=0  AutoFrameSizeCalculation=off
  GRANK : simulink/Logic and Bit Operations/Compare To Constant  Commented=on  relop===  const=3  OutDataTypeStr=boolean
  Goto106 : Goto  Commented=on  GotoTag=SI_b_GRANK
  Goto48 : Goto  Commented=on  GotoTag=SI_b_ACC
  Goto58 : Goto  Commented=on  GotoTag=SI_b_ON
  Goto69 : Goto  Commented=on  GotoTag=SI_b_IGN
  Ground : Ground
  Ground1 : Ground
  Logical Operator3 : Logic  Commented=on  Operator=OR  AllPortsSameDT=off  OutDataTypeStr=boolean
  "OFF " : simulink/Logic and Bit Operations/Compare To Constant  relop===  const=0  OutDataTypeStr=boolean
  ON : simulink/Logic and Bit Operations/Compare To Constant  Commented=on  relop===  const=2  OutDataTypeStr=boolean
  RLDoorRlsDriver : DoorRlsDriver/DoorRlsDriver  SystemSampleTime=-1  VariantActivationTime=update diagram  Latency=0  AutoFrameSizeCalculation=off
  RLDoorRlsReq : DoorRlsReq/DoorRlsReq  SystemSampleTime=-1  VariantActivationTime=update diagram  Latency=0  AutoFrameSizeCalculation=off
  Recycle Bin : Subsystem
  Terminator{,1..10,15,17} (13 alike) : Terminator
  VbOUT_REL_FLLockReleaseInsdSW_flg : Outport
  VbOUT_REL_FLLockReleaseOutsdSW_flg : Outport  Port=2
  VbOUT_REL_FLDoorOpenSwitch_flg : Outport  Port=3
  VbOUT_REL_FLDoorAjarSwitch_flg : Outport  Port=4
  VeOUT_REL_FLReleaseLatchStatus_sig : Outport  Port=5
  VbOUT_REL_RLLockReleaseInsdSW_flg : Outport  Port=6
  VbOUT_REL_RLLockReleaseOutsdSW_flg : Outport  Port=7
  VbOUT_REL_RLDoorOpenSwitch_flg : Outport  Port=8
  VbOUT_REL_RLDoorAjarSwitch_flg : Outport  Port=9
  VeOUT_REL_RLChildrenProtectSwitch_sig : Outport  Port=10
  VeOUT_REL_RLReleaseLatchStatus_sig : Outport  Port=11
  VeOUT_REL_HandleSwitchStsFL_sig : Outport  Port=12
  VeOUT_REL_HandleSwitchStsRR_sig : Outport  Port=13
  VbOUT_REL_FLDoorMotorA_flg : Outport  Port=14
  VbOUT_REL_FLDoorMotorB_flg : Outport  Port=15
  VbOUT_REL_RLDoorMotorA_flg : Outport  Port=16
  VbOUT_REL_RLDoorMotorB_flg : Outport  Port=17
  wires:
  "OFF "/1 -> [SI_b_OFF]
  [SI_PowerMode] -> "OFF "/1, GRANK/1, ON/1, ACC/1
  ON/1 -> Goto58/1, Logical Operator3/1
  GRANK/1 -> Goto106/1, Logical Operator3/2
  Logical Operator3/1 -> Goto69/1
  ACC/1 -> Goto48/1
  FLDoorRlsDriver/2 -> [SO_b_FLDoorMotorB]
  FLDoorRlsDriver/1 -> [SO_b_FLDoorMotorA]
  [SO_b_FLDoorRlsReq] -> FLDoorRlsDriver/1
  [SI_b_FLDoorAjar] -> FLDoorRlsDriver/2
  [SI_b_FLCinchHome] -> FLDoorRlsDriver/4
  [SI_b_ElecDoorCfg] -> FLDoorRlsDriver/5
  FLDoorRlsDriver/3 -> [SO_e_FLDoorMotorCmd]
  FLDoorRlsDriver/4 -> Terminator/1
  RLDoorRlsDriver/5 -> Terminator2/1
  [SI_b_FLDoorOpen] -> FLDoorRlsDriver/3
  FLDoorRlsReq/1 -> [SO_b_FLDoorRlsReq]
  RLDoorRlsReq/1 -> [SO_b_RLDoorRlsReq]
  FLDoorRlsDriver/5 -> Terminator15/1
  [SO_b_RLDoorRlsReq] -> RLDoorRlsDriver/1
  [SI_b_RLDoorAjar] -> RLDoorRlsDriver/2
  [SI_b_RLDoorOpen] -> RLDoorRlsDriver/3
  [SI_b_RLCinchHome] -> RLDoorRlsDriver/4
  [SI_b_ElecDoorCfg] -> RLDoorRlsDriver/5
  RLDoorRlsDriver/1 -> [SO_b_RLDoorMotorA]
  RLDoorRlsDriver/3 -> [SO_e_RLDoorMotorCmd]
  RLDoorRlsDriver/2 -> [SO_b_RLDoorMotorB]
  RLDoorRlsDriver/4 -> Terminator17/1
  [SO_b_FLDoorHndBtnSts] -> FLDoorRlsReq/9
  [SI_b_OFF] -> FLDoorRlsReq/1
  [SI_e_EspVehSpd] -> FLDoorRlsReq/2
  [SI_b_EspVehSpdVld] -> FLDoorRlsReq/3
  [SI_m_VcuGearPosn] -> FLDoorRlsReq/4
  [SI_m_DrvDoorLockSts] -> FLDoorRlsReq/5
  [SO_m_FLDoorRatSts] -> FLDoorRlsReq/6
  [SO_b_FLDoorInBtnSts] -> FLDoorRlsReq/7
  [SI_b_OFF] -> RLDoorRlsReq/1
  [SI_e_EspVehSpd] -> RLDoorRlsReq/2
  [SI_b_EspVehSpdVld] -> RLDoorRlsReq/3
  [SI_m_VcuGearPosn] -> RLDoorRlsReq/4
  [SO_b_RLDoorHndBtnSts] -> RLDoorRlsReq/9
  [SI_m_PassDoorLockSts] -> RLDoorRlsReq/5
  [SO_m_RLDoorRatSts] -> RLDoorRlsReq/6
  [SO_b_RLDoorInBtnSts] -> RLDoorRlsReq/7
  DoorSwSts/1(SL_b_FLDoorInBtnSts) -> [SO_b_FLDoorInBtnSts]
  [SI_b_FLDoorInBtn] -> DoorSwSts/2(SI_b_FLDoorInBtn)
  [SI_b_CrashSts] -> DoorSwSts/1(SI_b_CrashSts)
  [SI_b_RLDoorInBtn] -> DoorSwSts/3(SI_b_RLDoorInBtn)
  [SI_b_FLDoorHndBtn] -> DoorSwSts/4(SI_b_FLDoorHndBtn)
  [SI_b_RLDoorHndBtn] -> DoorSwSts/5(SI_b_RLDoorHndBtn)
  DoorSwSts/2(SL_b_RLDoorInBtnSts) -> [SO_b_RLDoorInBtnSts]
  DoorSwSts/3(SL_b_FLDoorHndBtnSts) -> [SO_b_FLDoorHndBtnSts]
  DoorSwSts/4(SL_b_RLDoorHndBtnSts) -> [SO_b_RLDoorHndBtnSts]
  [SI_b_CentFLDoorBtnSts] -> FLDoorRlsReq/11
  [SI_b_CentAllDoorBtnSts] -> FLDoorRlsReq/12
  Constant7/1 -> FLDoorRlsReq/13
  [SI_m_FLDoorHandPosSts] -> FLDoorRlsReq/10
  [SI_b_CentAllDoorBtnSts] -> RLDoorRlsReq/12
  [SI_m_RLDoorHandPosSts] -> RLDoorRlsReq/10
  [SI_b_CentRLDoorBtnSts] -> RLDoorRlsReq/11
  [SI_b_RLChildLckSts] -> RLDoorRlsReq/13
  Constant10/1 -> RLDoorRlsReq/14
  [SL_e_FLDoorRlsDelayTime] -> FLDoorRlsDriver/6
  [SL_e_RLDoorRlsDelayTime] -> RLDoorRlsDriver/6
  Constant6/1 -> RLDoorRlsReq/15
  Constant/1 -> Data Store Write/1
  FLDoorRlsReq/2 -> [SL_e_FLDoorRlsDelayTime]
  FLDoorRlsReq/3 -> Terminator1/1
  RLDoorRlsReq/2 -> [SL_e_RLDoorRlsDelayTime]
  RLDoorRlsReq/3 -> Terminator3/1
  [SO_m_FLDoorRatSts] -> Data Type Conversion3/1
  [SO_m_RLDoorRatSts] -> Data Type Conversion6/1
  DoorRatSts/1(SO_m_FLDoorRatSts) -> [SO_m_FLDoorRatSts]
  DoorRatSts/2(SO_m_RLDoorRatSts) -> [SO_m_RLDoorRatSts]
  [SO_e_FLDoorMotorCmd] -> Data Type Conversion8/1
  [SO_e_RLDoorMotorCmd] -> Data Type Conversion10/1
  Data Type Conversion12/1 -> [SI_m_DrvDoorLockSts]
  Data Type Conversion13/1 -> [SI_m_PassDoorLockSts]
  Data Type Conversion14/1 -> [SI_m_VcuGearPosn]
  Data Type Conversion15/1 -> [SI_m_FLDoorHandPosSts]
  Data Type Conversion17/1 -> [SI_m_RLDoorHandPosSts]
  [SI_b_FLDoorOpen] -> DoorRatSts/1(SI_b_FLDoorOpen)
  [SI_b_RLDoorOpen] -> DoorRatSts/3(SI_b_RLDoorOpen)
  [SI_b_FLDoorAjar] -> DoorRatSts/2(SI_b_FLDoorAjar)
  [SI_b_RLDoorAjar] -> DoorRatSts/4(SI_b_RLDoorAjar)
  VeINP_HWA_LRChildrenProtectSwitch_sig/1 -> [SI_b_RLChildLckSts]
  VbOUT_SP_FLDoorAjarSts_flg/1 -> [SI_b_FLDoorAjar]
  VbOUT_SP_RLDoorAjarSts_flg/1 -> [SI_b_RLDoorAjar]
  VbOUT_HWA_FLDoorFullOpen_flg/1 -> [SI_b_FLDoorOpen]
  VbOUT_HWA_RLDoorFullOpen_flg/1 -> [SI_b_RLDoorOpen]
  VeOUT_DLK_LHFDoorLockSts_sig/1 -> Data Type Conversion12/1
  VeOUT_DLK_LHRDoorLockSts_sig/1 -> Data Type Conversion13/1
  VeINP_CAN_PowerMode_sig/1 -> [SI_PowerMode]
  VbINP_HWA_FLDoorButton_flg/1 -> [SI_b_FLDoorInBtn]
  VbINP_HWA_RLDoorButton_flg/1 -> [SI_b_RLDoorInBtn]
  VbINP_HWA_FLDoorHandleSW_flg/1 -> [SI_b_FLDoorHndBtn]
  VbINP_HWA_RLDoorHandleSW_flg/1 -> [SI_b_RLDoorHndBtn]
  VmOUT_DLK_LockSrc_enum/1 -> Terminator8/1
  VbOUT_DLK_FLUnlock_flg/1 -> Terminator9/1
  VbOUT_DLK_RLUnlock_flg/1 -> Terminator4/1
  VeOUT_SP_EspVehSpd_kmh/1 -> [SI_e_EspVehSpd]
  VbINP_CAN_EspVehSpdVld_flg/1 -> [SI_b_EspVehSpdVld]
  VbOUT_SP_CrashOutpSts_flg/1 -> [SI_b_CrashSts]
  [SO_b_FLDoorRlsReq] -> Terminator5/1
  [SO_b_RLDoorRlsReq] -> Terminator6/1
  Constant1/1 -> [SI_b_ElecDoorCfg]
  Constant2/1 -> [SI_b_FLCinchHome]
  Constant3/1 -> [SI_b_RLCinchHome]
  [SO_b_FLDoorInBtnSts] -> VbOUT_REL_FLLockReleaseInsdSW_flg/1
  [SO_b_FLDoorHndBtnSts] -> VbOUT_REL_FLLockReleaseOutsdSW_flg/1
  [SI_b_FLDoorOpen] -> VbOUT_REL_FLDoorOpenSwitch_flg/1
  [SI_b_FLDoorAjar] -> VbOUT_REL_FLDoorAjarSwitch_flg/1
  Data Type Conversion8/1 -> VeOUT_REL_FLReleaseLatchStatus_sig/1
  [SO_b_RLDoorInBtnSts] -> VbOUT_REL_RLLockReleaseInsdSW_flg/1
  [SO_b_RLDoorHndBtnSts] -> VbOUT_REL_RLLockReleaseOutsdSW_flg/1
  [SI_b_RLDoorOpen] -> VbOUT_REL_RLDoorOpenSwitch_flg/1
  [SI_b_RLDoorAjar] -> VbOUT_REL_RLDoorAjarSwitch_flg/1
  [SI_b_RLChildLckSts] -> VeOUT_REL_RLChildrenProtectSwitch_sig/1
  Data Type Conversion10/1 -> VeOUT_REL_RLReleaseLatchStatus_sig/1
  Ground/1 -> VeOUT_REL_HandleSwitchStsFL_sig/1
  Ground1/1 -> VeOUT_REL_HandleSwitchStsRR_sig/1
  [SO_b_RLDoorMotorB] -> VbOUT_REL_RLDoorMotorB_flg/1
  [SO_b_RLDoorMotorA] -> VbOUT_REL_RLDoorMotorA_flg/1
  [SO_b_FLDoorMotorA] -> VbOUT_REL_FLDoorMotorA_flg/1
  [SO_b_FLDoorMotorB] -> VbOUT_REL_FLDoorMotorB_flg/1
  Data Type Conversion3/1 -> Terminator7/1
  Data Type Conversion6/1 -> Terminator10/1

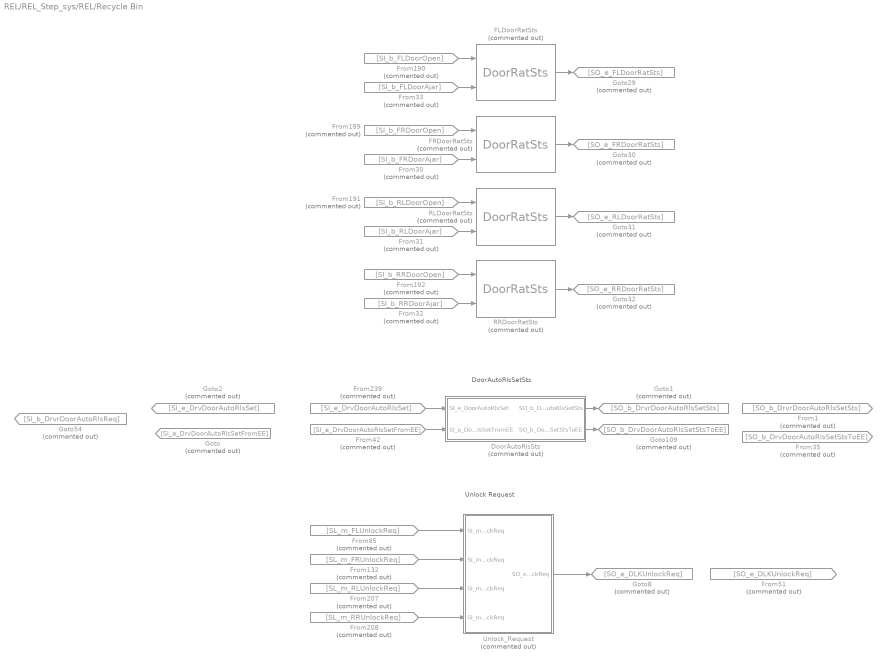
== system REL/REL_Step_sys/REL/Recycle Bin ==
  note: DoorAutoRlsSetSts
  note: Unlock Request
  DoorAutoRlsSts : Stateflow chart  Commented=on  TreatAsAtomicUnit=on
  FLDoorRatSts : DoorRatSts/DoorRatSts  Commented=on  SystemSampleTime=-1  VariantActivationTime=update diagram  Latency=0  AutoFrameSizeCalculation=off
  FRDoorRatSts : DoorRatSts/DoorRatSts  Commented=on  SystemSampleTime=-1  VariantActivationTime=update diagram  Latency=0  AutoFrameSizeCalculation=off
  From1 : From  Commented=on  GotoTag=SO_b_DrvrDoorAutoRlsSetSts
  From132 : From  Commented=on  GotoTag=SL_m_FRUnlockReq
  From189 : From  Commented=on  GotoTag=SI_b_FRDoorOpen
  From190 : From  Commented=on  GotoTag=SI_b_FLDoorOpen
  From191 : From  Commented=on  GotoTag=SI_b_RLDoorOpen
  From192 : From  Commented=on  GotoTag=SI_b_RRDoorOpen
  From207 : From  Commented=on  GotoTag=SL_m_RLUnlockReq
  From208 : From  Commented=on  GotoTag=SL_m_RRUnlockReq
  From239 : From  Commented=on  GotoTag=SI_e_DrvDoorAutoRlsSet
  From30 : From  Commented=on  GotoTag=SI_b_FRDoorAjar
  From31 : From  Commented=on  GotoTag=SI_b_RLDoorAjar
  From32 : From  Commented=on  GotoTag=SI_b_RRDoorAjar
  From33 : From  Commented=on  GotoTag=SI_b_FLDoorAjar
  From35 : From  Commented=on  GotoTag=SO_b_DrvDoorAutoRlsSetStsToEE
  From42 : From  Commented=on  GotoTag=SI_e_DrvDoorAutoRlsSetFromEE
  From51 : From  Commented=on  GotoTag=SO_e_DLKUnlockReq
  From85 : From  Commented=on  GotoTag=SL_m_FLUnlockReq
  Goto : Goto  Commented=on  GotoTag=SI_e_DrvDoorAutoRlsSetFromEE
  Goto1 : Goto  Commented=on  GotoTag=SO_b_DrvrDoorAutoRlsSetSts
  Goto109 : Goto  Commented=on  GotoTag=SO_b_DrvDoorAutoRlsSetStsToEE
  Goto2 : Goto  Commented=on  GotoTag=SI_e_DrvDoorAutoRlsSet
  Goto29 : Goto  Commented=on  GotoTag=SO_e_FLDoorRatSts
  Goto30 : Goto  Commented=on  GotoTag=SO_e_FRDoorRatSts
  Goto31 : Goto  Commented=on  GotoTag=SO_e_RLDoorRatSts
  Goto32 : Goto  Commented=on  GotoTag=SO_e_RRDoorRatSts
  Goto54 : Goto  Commented=on  GotoTag=SI_b_DrvrDoorAutoRlsReq
  Goto8 : Goto  Commented=on  GotoTag=SO_e_DLKUnlockReq
  RLDoorRatSts : DoorRatSts/DoorRatSts  Commented=on  SystemSampleTime=-1  VariantActivationTime=update diagram  Latency=0  AutoFrameSizeCalculation=off
  RRDoorRatSts : DoorRatSts/DoorRatSts  Commented=on  SystemSampleTime=-1  VariantActivationTime=update diagram  Latency=0  AutoFrameSizeCalculation=off
  Unlock_Request : Stateflow chart  Commented=on  TreatAsAtomicUnit=on
  wires:
  FLDoorRatSts/1 -> Goto29/1
  From191/1 -> RLDoorRatSts/1
  FRDoorRatSts/1 -> Goto30/1
  From190/1 -> FLDoorRatSts/1
  From192/1 -> RRDoorRatSts/1
  From189/1 -> FRDoorRatSts/1
  RRDoorRatSts/1 -> Goto32/1
  RLDoorRatSts/1 -> Goto31/1
  From30/1 -> FRDoorRatSts/2
  From32/1 -> RRDoorRatSts/2
  From31/1 -> RLDoorRatSts/2
  From33/1 -> FLDoorRatSts/2
  DoorAutoRlsSts/1(SO_b_DoorAutoRlsSetSts) -> Goto1/1
  DoorAutoRlsSts/2(SO_b_DoorAutoRlsSetStsToEE) -> Goto109/1
  From42/1 -> DoorAutoRlsSts/2(SI_e_DoorAutoRlsSetFromEE)
  From239/1 -> DoorAutoRlsSts/1(SI_e_DoorAutoRlsSet)
  From132/1 -> Unlock_Request/2(SI_m_FRUnlockReq)
  From208/1 -> Unlock_Request/4(SI_m_RRUnlockReq)
  From207/1 -> Unlock_Request/3(SI_m_RLUnlockReq)
  Unlock_Request/1(SO_e_UnlockReq) -> Goto8/1
  From85/1 -> Unlock_Request/1(SI_m_FLUnlockReq)

== stateflow chart REL/REL_Step_sys/REL/Recycle Bin/DoorAutoRlsSts ==
  state DoorLockSet
    (default) -> (junction 127) : /* DoorLockSet */
    DoorLockSet -> (junction 127)
    (junction 127) -> (junction 128) [order 1] : [SI_e_DoorAutoRlsSet == 1 || ...
        | (SI_e_DoorAutoRlsSet != 2 && SL_e_DoorAutoRlsSetBackup == 1)]
    (junction 127) -> (junction 129) [order 2]
    (junction 128) -> (junction 136) : {SO_b_DoorAutoRlsSetSts = 1; ...
        | SO_b_DoorAutoRlsSetStsToEE = 1; ...
        | SL_e_DoorAutoRlsSetBackup = 1}
    (junction 129) -> (junction 130) [order 1] : [SI_e_DoorAutoRlsSet == 2 || ...
        | (SI_e_DoorAutoRlsSet != 1 && SL_e_DoorAutoRlsSetBackup == 2)]
    (junction 129) -> (junction 131) [order 2]
    (junction 130) -> (junction 135) : {SO_b_DoorAutoRlsSetSts = 0; ...
        | SO_b_DoorAutoRlsSetStsToEE = 0; ...
        | SL_e_DoorAutoRlsSetBackup = 2}
    (junction 131) -> (junction 132) [order 1] : [SI_e_DoorAutoRlsSetFromEE == 1]
    (junction 131) -> (junction 151) [order 2]
    (junction 132) -> (junction 134) : {SO_b_DoorAutoRlsSetSts = 1; ...
        | SO_b_DoorAutoRlsSetStsToEE = 1;}
    (junction 151) -> (junction 159) [order 1] : [SI_e_DoorAutoRlsSetFromEE == 0]
    (junction 151) -> (junction 133) [order 2]
    (junction 159) -> (junction 160) : {SO_b_DoorAutoRlsSetSts = 0; ...
        | SO_b_DoorAutoRlsSetStsToEE = 0;}
    (junction 160) -> (junction 133)
    (junction 134) -> (junction 160)
    (junction 135) -> (junction 134)
    (junction 136) -> (junction 135)
    (junction 133) -> (junction 137)
  data: SO_b_DoorAutoRlsSetSts output boolean; SI_e_DoorAutoRlsSet input uint8; SI_e_DoorAutoRlsSetFromEE input uint8; SO_b_DoorAutoRlsSetStsToEE output boolean; SL_e_DoorAutoRlsSetBackup local uint8 =0

== stateflow chart REL/REL_Step_sys/REL/Recycle Bin/Unlock_Request ==
  state req = GetDrvUnlockReq [function]
    (default) -> (junction 216)
    (junction 216) -> (junction 217) [order 1] : [SI_m_FLUnlockReq == Unlock_PE]
    (junction 216) -> (junction 218) [order 2]
    (junction 217) -> (junction 222) : {req = Unlock_PE;}
    (junction 218) -> (junction 219) [order 1] : [SI_m_FLUnlockReq == Unlock_Req]
    (junction 218) -> (junction 220) [order 2] : {req = Unlock_Idle;}
    (junction 219) -> (junction 221) : {req = Unlock_Req;}
    (junction 221) -> (junction 220)
    (junction 222) -> (junction 221)
    (junction 220) -> (junction 223)
  state UnlockReq
    (default) -> (junction 185)
    UnlockReq -> (junction 185)
    (junction 185) -> (junction 186) [order 1] : [(GetDrvUnlockReq() == Unlock_Req && GetPassUnlockReq() == Unlock_Req) || ...
        | GetDrvUnlockReq() == Unlock_PE || ...
        | GetPassUnlockReq() == Unlock_PE]
    (junction 185) -> (junction 187) [order 2]
    (junction 186) -> (junction 194) : {SO_e_UnlockReq = 3;}
    (junction 187) -> (junction 188) [order 1] : [GetDrvUnlockReq() == Unlock_Idle && ...
        | GetPassUnlockReq() == Unlock_Req]
    (junction 187) -> (junction 189) [order 2]
    (junction 188) -> (junction 193) : {SO_e_UnlockReq = 2;}
    (junction 189) -> (junction 190) [order 1] : [GetDrvUnlockReq() == Unlock_Req && ...
        | GetPassUnlockReq() == Unlock_Idle]
    (junction 189) -> (junction 191) [order 2] : {SO_e_UnlockReq = 0;}
    (junction 190) -> (junction 192) : {SO_e_UnlockReq = 1;}
    (junction 192) -> (junction 191)
    (junction 193) -> (junction 192)
    (junction 194) -> (junction 193)
    (junction 191) -> (junction 195)
  state req = GetPassUnlockReq [function]
    (default) -> (junction 232)
    (junction 232) -> (junction 228) [order 1] : [SI_m_FRUnlockReq == Unlock_PE || ...
        | SI_m_RLUnlockReq == Unlock_PE || ...
        | SI_m_RRUnlockReq == Unlock_PE]
    (junction 232) -> (junction 234) [order 2]
    (junction 228) -> (junction 238) : {req = Unlock_PE;}
    (junction 234) -> (junction 237) [order 1] : [SI_m_FRUnlockReq == Unlock_Req || ...
        | SI_m_RLUnlockReq == Unlock_Req || ...
        | SI_m_RRUnlockReq == Unlock_Req]
    (junction 234) -> (junction 240) [order 2] : {req = Unlock_Idle;}
    (junction 237) -> (junction 241) : {req = Unlock_Req;}
    (junction 241) -> (junction 240)
    (junction 238) -> (junction 241)
    (junction 240) -> (junction 239)
  data: req function_output double; req function_output double; SO_e_UnlockReq output uint8; SI_m_FLUnlockReq input Enum: Unlock_Req_E; SI_m_FRUnlockReq input Enum: Unlock_Req_E; SI_m_RLUnlockReq input Enum: Unlock_Req_E; SI_m_RRUnlockReq input Enum: Unlock_Req_E

== stateflow chart REL/REL_Step_sys/REL/DoorRatSts ==
  state DoorRatSts
    (default) -> (junction 42)
    DoorRatSts -> (junction 42)
    (junction 42) -> (junction 53) : {SO_m_FLDoorRatSts = GetDoorRatSts(SI_b_FLDoorAjar, SI_b_FLDoorOpen)}
    (junction 53) -> (junction 45)
    (junction 45) -> (junction 48)
    (junction 48) -> (junction 55)
    (junction 55) -> (junction 57) : {SO_m_RLDoorRatSts = GetDoorRatSts(SI_b_RLDoorAjar, SI_b_RLDoorOpen)}
    (junction 57) -> (junction 58)
    (junction 58) -> (junction 59)
    (junction 59) -> (junction 56)
  state status = GetDoorRatSts(ajar, open) [function]
    (default) -> (junction 24)
    (junction 24) -> (junction 25) [order 1] : [ajar == 0 && open == 0]
    (junction 24) -> (junction 26) [order 2]
    (junction 25) -> (junction 33) : {status = Rat_All_Lock;}
    (junction 26) -> (junction 27) [order 1] : [ajar == 1 && open ==0]
    (junction 26) -> (junction 28) [order 2]
    (junction 27) -> (junction 32) : {status = Rat_Half_Lock;}
    (junction 28) -> (junction 29) [order 1] : [ajar == 1 && open == 1]
    (junction 28) -> (junction 30) [order 2] : {status = Rat_Invalid;}
    (junction 29) -> (junction 31) : {status = Rat_Unlock;}
    (junction 31) -> (junction 30)
    (junction 32) -> (junction 31)
    (junction 33) -> (junction 32)
    (junction 30) -> (junction 34)
  data: ajar function_input double; open function_input double; status function_output double; SI_b_FLDoorOpen input boolean; SO_m_FLDoorRatSts output Enum: Rat_Sts_E; SI_b_FLDoorAjar input boolean; SO_m_RLDoorRatSts output Enum: Rat_Sts_E; SI_b_RLDoorOpen input boolean; SI_b_RLDoorAjar input boolean

== stateflow chart REL/REL_Step_sys/REL/DoorSwSts ==
  state NoCrash
    en,du:
    SL_b_FLDoorInBtnSts = SI_b_FLDoorInBtn;
    SL_b_RLDoorInBtnSts = SI_b_RLDoorInBtn;
    SL_b_FLDoorHndBtnSts = SI_b_FLDoorHndBtn;
    SL_b_RLDoorHndBtnSts = SI_b_RLDoorHndBtn;
  state Crash
    en,du:
    SL_b_FLDoorInBtnSts = 0;
    SL_b_RLDoorInBtnSts = 0;
    SL_b_FLDoorHndBtnSts = 0;
    SL_b_RLDoorHndBtnSts = 0;
  (default) -> NoCrash
  NoCrash -> Crash : [hasChangedTo(SI_b_CrashSts, 1)]
  Crash -> NoCrash : [after(600, tick)]
  data: SL_b_FLDoorInBtnSts output boolean; SI_b_CrashSts input boolean; SI_b_FLDoorInBtn input boolean; SI_b_RLDoorInBtn input boolean; SL_b_RLDoorInBtnSts output boolean; SI_b_FLDoorHndBtn input boolean; SI_b_RLDoorHndBtn input boolean; SL_b_FLDoorHndBtnSts output boolean; SL_b_RLDoorHndBtnSts output boolean
